simulink model "procesor"  (R2020a)
settings: Solver=VariableStepAuto  StartTime=0.0  StopTime=inf  RelTol=1e-3
libraries: simulink_extras x40, commutil2 x3
settings Model: NumberOfSteps=3  EnablePacing=on  Creator=BakuTer  LastModifiedBy=BakuTer
settings ModelReferenceCC: UpdateModelReferenceTargets=AssumeUpToDate

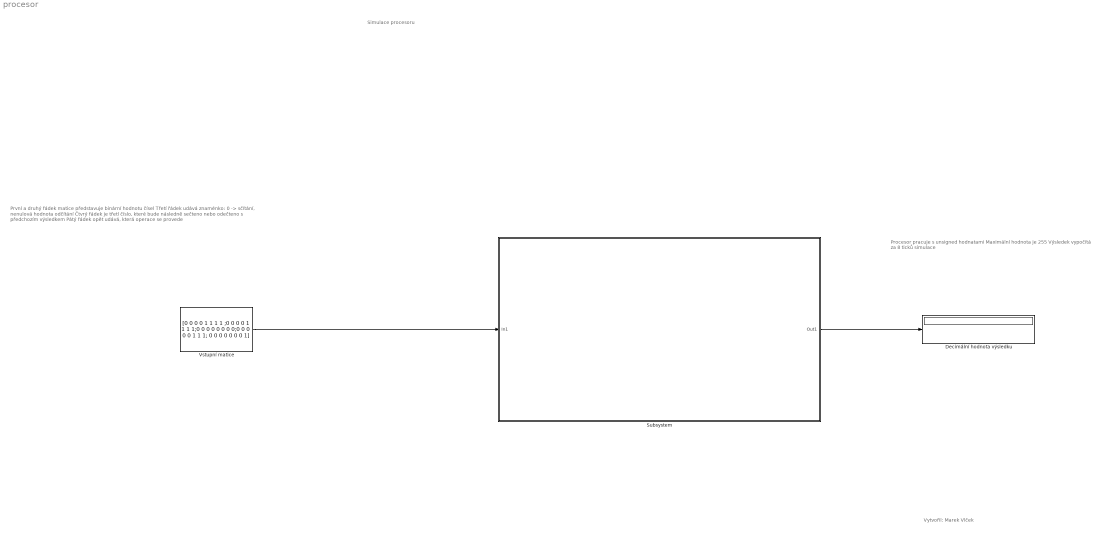
== system procesor ==
  note: Vytvořil: Marek Vlček
  note: Simulace procesoru
  note: Procesor pracuje s unsigned hodnatami
      |
      | Maximální hodnota je 255
      |
      | Výsledek vypočítá za 8 ticků simulace
  note: První a druhý řádek matice představuje binární hodnotu čísel
      |
      | Třetí řádek udává znaménko: 0 -> sčítání, nenulová hodnota odčítání
      |
      | Čtvrý řádek je třetí číslo, které bude následně sečteno nebo odečteno s předchozím výsledkem
      |
      | Pátý řádek opět udává, která operace se provede
  Decimální hodnota výsledku : Display
  Subsystem : Subsystem
      mask Display: image('T:\Stažené Soubory\jak-vybrat-procesor.jpg'); % Use "Edit Image" on toolstrip to change.
  Vstupní matice : Constant  Value=[0 0 0 0 1 1 1 1 ;0 0 0 0 1 1 1 1;0 0 0 0 0 0 0 0;0 0 0 0 0 1 1 1; 0 0 0 0 0 0 0 1]  VectorParams1D=off
  wires:
  Vstupní matice/1 -> Subsystem/1(In1)
  Subsystem/1(Out1) -> Decimální hodnota výsledku/1

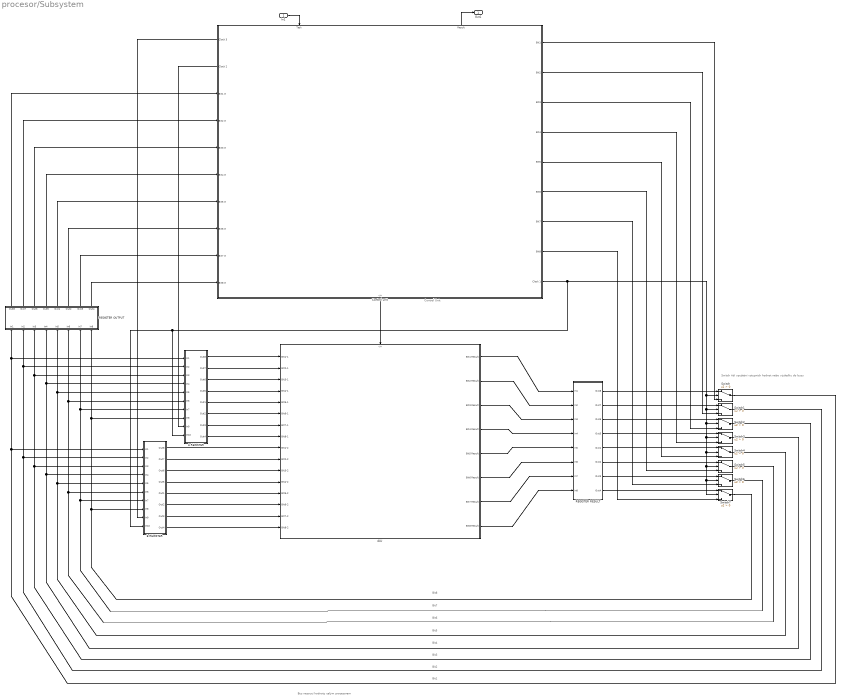
== system procesor/Subsystem ==
  note: Switch řídí vpuštění vstupních hodnot nebo výsledku do busu
  note: Bus nesoucí hodnoty celým procesorem
  note: Bit1
  note: Control Unit
  note: Bit2
  note: Bit3
  note: Bit4
  note: Bit5
  note: Bit6
  note: Bit7
  note: Bit8
  In1 : Inport
  "A REGISTER " : Subsystem
  ALU : Subsystem
      settings: PortSchema="{\"entries\":[{\"content\":{\"sides\":[{\"content\":{\"connectorIds\":[\"In1\",\"In2\",\"In3\",\"In4\",\"In5\",\"In6\",\"In7\",\"In8\",\"In9\",\"In10\",\"In11\",\"In12\",\"In13\",\"In14\",\"In15\",\"In16\"]},\"type\":\"ConnectorPlacement.EquallySpacedRectSide\",\"uuid\":\"ebc9eafb-b3d6-44c3-afac-e365ab2b3d65\"},{\"content\":{\"connectorIds\":[\"Out1\",\"Out2\",\"Out3\",\"Out4\",\"Out5\",\"Out6\",\"Out7\",\"Out8\"],\"side\":\"RIGHT\"},\"type\":\"ConnectorPlacement.EquallySpacedRectSide\",\"uuid\":\"9653c2f1-04bb-448f-a78f-504bc47adb0d\"},{\"content\":{\"connectorIds\":[\"In17\"],\"side\":\"TOP\"},\"type\":\"ConnectorPlacement.EquallySpacedRectSide\",\"uuid\":\"4b4c1363-efa0-4666-9ae9-c7b80d9168bd\"}]},\"type\":\"ConnectorPlacement.EquallySpacedConnector\",\"uuid\":\"b9b0fe66-7efa-45ab-a891-884508afc9d3\"}],\"packageUris\":[\"http://schema.mathworks.com/mf0/Connector/19700101\"],\"version\":\"1.0\"}"
  "B REGISTER " : Subsystem
  Control unit : Subsystem
      settings: PortSchema="{\"entries\":[{\"content\":{\"sides\":[{\"content\":{\"connectorIds\":[\"Out12\",\"Out13\",\"In1\",\"In2\",\"In3\",\"In4\",\"In5\",\"In6\",\"In7\",\"In8\"]},\"type\":\"ConnectorPlacement.EquallySpacedRectSide\",\"uuid\":\"83bcb533-41cd-4a45-82b0-e1e863155d62\"},{\"content\":{\"connectorIds\":[\"Out1\",\"Out2\",\"Out3\",\"Out4\",\"Out5\",\"Out6\",\"Out7\",\"Out8\",\"Out9\"],\"side\":\"RIGHT\"},\"type\":\"ConnectorPlacement.EquallySpacedRectSide\",\"uuid\":\"5279903c-db3c-41cc-9a95-b325bef2964f\"},{\"content\":{\"connectorIds\":[\"In9\",\"Out11\"],\"side\":\"TOP\"},\"type\":\"ConnectorPlacement.EquallySpacedRectSide\",\"uuid\":\"7ad9fff0-61c8-4fe7-a492-4231851eacd1\"},{\"content\":{\"connectorIds\":[\"Out10\"],\"side\":\"BOTTOM\"},\"type\":\"ConnectorPlacement.EquallySpacedRectSide\",\"uuid\":\"4f77aa59-d7ef-4985-b89c-d7e6d2465284\"}]},\"type\":\"ConnectorPlacement.EquallySpacedConnector\",\"uuid\":\"61151066-d116-425f-b948-57ee4dd34c87\"}],\"packageUris\":[\"http://schema.mathworks.com/mf0/Connector/19700101\"],\"version\":\"1.0\"}"
  REGISTER OUTPUT : Subsystem
  "REGISTER RESULT " : Subsystem
  Switch{,1..7} (8 alike) : Switch  Criteria=u2 > Threshold
  Out1 : Outport
  wires:
  Control unit/9(Clock 1) -> Switch2/2, Switch7/2, Switch6/2, Switch5/2, Switch4/2, Switch3/2, Switch1/2, Switch/2, "A REGISTER "/10(In10), "B REGISTER "/10(In10)
  ALU/7(Bit7 Result) -> "REGISTER RESULT "/7(In7)
  Switch2/1 -> "B REGISTER "/3(In3), REGISTER OUTPUT/3(In3), "A REGISTER "/3(In3)
  Control unit/8(Bit8) -> Switch7/3
  REGISTER OUTPUT/4(Out5) -> Control unit/4(Bit4 in)
  ALU/8(Bit8 Result) -> "REGISTER RESULT "/8(In8)
  "A REGISTER "/4(Out5) -> ALU/4(Bit4-1)
  REGISTER OUTPUT/7(Out3) -> Control unit/7(Bit7 in)
  Switch7/1 -> REGISTER OUTPUT/8(In8), "A REGISTER "/8(In8), "B REGISTER "/8(In8)
  "A REGISTER "/3(Out6) -> ALU/3(Bit3-1)
  "REGISTER RESULT "/6(Out2) -> Switch5/1
  ALU/1(Bit1 Result) -> "REGISTER RESULT "/1(In1)
  REGISTER OUTPUT/3(Out6) -> Control unit/3(Bit3 in)
  "B REGISTER "/5(Out1) -> ALU/13(Bit5-2)
  "A REGISTER "/2(Out7) -> ALU/2(Bit2-1)
  "REGISTER RESULT "/3(Out6) -> Switch2/1
  ALU/4(Bit4 Result) -> "REGISTER RESULT "/4(In4)
  "REGISTER RESULT "/4(Out5) -> Switch3/1
  "A REGISTER "/7(Out3) -> ALU/7(Bit7-1)
  "B REGISTER "/1(Out8) -> ALU/9(Bit1-2)
  Switch/1 -> REGISTER OUTPUT/1(In1), "A REGISTER "/1(In1), "B REGISTER "/1(In1)
  Control unit/2(Bit2) -> Switch1/3
  "B REGISTER "/3(Out6) -> ALU/11(Bit3-2)
  "REGISTER RESULT "/7(Out3) -> Switch6/1
  "A REGISTER "/1(Out8) -> ALU/1(Bit1-1)
  Switch1/1 -> REGISTER OUTPUT/2(In2), "A REGISTER "/2(In2), "B REGISTER "/2(In2)
  ALU/2(Bit2 Result) -> "REGISTER RESULT "/2(In2)
  "REGISTER RESULT "/1(Out8) -> Switch/1
  ALU/6(Bit6 Result) -> "REGISTER RESULT "/6(In6)
  "B REGISTER "/6(Out2) -> ALU/14(Bit6-2)
  "B REGISTER "/8(Out4) -> ALU/16(Bit8-2)
  "B REGISTER "/7(Out3) -> ALU/15(Bit7-2)
  "A REGISTER "/8(Out4) -> ALU/8(Bit8-1)
  ALU/3(Bit3 Result) -> "REGISTER RESULT "/3(In3)
  Switch5/1 -> REGISTER OUTPUT/6(In6), "A REGISTER "/6(In6), "B REGISTER "/6(In6)
  "REGISTER RESULT "/8(Out4) -> Switch7/1
  Control unit/5(Bit5) -> Switch4/3
  "A REGISTER "/6(Out2) -> ALU/6(Bit6-1)
  REGISTER OUTPUT/2(Out7) -> Control unit/2(Bit2 in)
  Switch3/1 -> "B REGISTER "/4(In4), "A REGISTER "/4(In4), REGISTER OUTPUT/4(In4)
  "B REGISTER "/2(Out7) -> ALU/10(Bit2-2)
  Control unit/1(Bit1) -> Switch/3
  Control unit/3(Bit3) -> Switch2/3
  Switch6/1 -> REGISTER OUTPUT/7(In7), "A REGISTER "/7(In7), "B REGISTER "/7(In7)
  ALU/5(Bit5 Result) -> "REGISTER RESULT "/5(In5)
  REGISTER OUTPUT/6(Out2) -> Control unit/6(Bit6 in)
  "REGISTER RESULT "/5(Out1) -> Switch4/1
  Control unit/7(Bit7) -> Switch6/3
  Switch4/1 -> REGISTER OUTPUT/5(In5), "A REGISTER "/5(In5), "B REGISTER "/5(In5)
  Control unit/4(Bit4) -> Switch3/3
  REGISTER OUTPUT/1(Out8) -> Control unit/1(Bit1 in)
  In1/1 -> Control unit/9(Task)
  "REGISTER RESULT "/2(Out7) -> Switch1/1
  REGISTER OUTPUT/5(Out1) -> Control unit/5(Bit5 in)
  Control unit/6(Bit6) -> Switch5/3
  Control unit/10(-/+) -> ALU/17(-/+)
  REGISTER OUTPUT/8(Out4) -> Control unit/8(Bit8 in)
  "B REGISTER "/4(Out5) -> ALU/12(Bit4-2)
  Control unit/13(Clock 2) -> "A REGISTER "/9(In9)
  Control unit/12(Clock 3) -> "B REGISTER "/9(In9)
  "A REGISTER "/5(Out1) -> ALU/5(Bit5-1)
  Control unit/11(Result) -> Out1/1

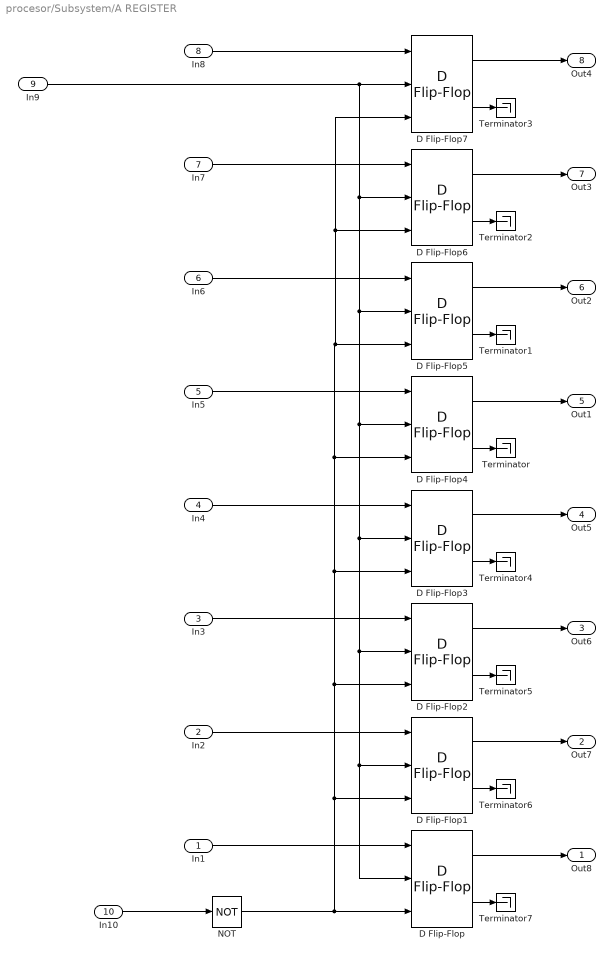
== system procesor/Subsystem/A REGISTER  ==
  In1 : Inport
  In2 : Inport  Port=2
  In3 : Inport  Port=3
  In4 : Inport  Port=4
  In5 : Inport  Port=5
  In6 : Inport  Port=6
  In7 : Inport  Port=7
  In8 : Inport  Port=8
  In9 : Inport  Port=9
  In10 : Inport  Port=10
  D Flip-Flop{,1..7} (8 alike) : simulink_extras/Flip Flops/D Flip-Flop
  NOT : Logic  Operator=NOT  IconShape=distinctive  AllPortsSameDT=off  OutDataTypeStr=boolean
  Terminator{,1..7} (8 alike) : Terminator
  Out8 : Outport
  Out7 : Outport  Port=2
  Out6 : Outport  Port=3
  Out5 : Outport  Port=4
  Out1 : Outport  Port=5
  Out2 : Outport  Port=6
  Out3 : Outport  Port=7
  Out4 : Outport  Port=8
  wires:
  D Flip-Flop5/2 -> Terminator1/1
  D Flip-Flop4/2 -> Terminator/1
  D Flip-Flop5/1 -> Out2/1
  D Flip-Flop3/2 -> Terminator4/1
  In1/1 -> D Flip-Flop/1
  D Flip-Flop6/2 -> Terminator2/1
  D Flip-Flop6/1 -> Out3/1
  D Flip-Flop/1 -> Out8/1
  D Flip-Flop7/2 -> Terminator3/1
  D Flip-Flop2/2 -> Terminator5/1
  D Flip-Flop1/2 -> Terminator6/1
  D Flip-Flop/2 -> Terminator7/1
  D Flip-Flop1/1 -> Out7/1
  D Flip-Flop4/1 -> Out1/1
  D Flip-Flop7/1 -> Out4/1
  In5/1 -> D Flip-Flop4/1
  In3/1 -> D Flip-Flop2/1
  In2/1 -> D Flip-Flop1/1
  In8/1 -> D Flip-Flop7/1
  In6/1 -> D Flip-Flop5/1
  In7/1 -> D Flip-Flop6/1
  In4/1 -> D Flip-Flop3/1
  In9/1 -> D Flip-Flop7/2, D Flip-Flop6/2, D Flip-Flop5/2, D Flip-Flop4/2, D Flip-Flop3/2, D Flip-Flop2/2, D Flip-Flop1/2, D Flip-Flop/2
  D Flip-Flop2/1 -> Out6/1
  D Flip-Flop3/1 -> Out5/1
  In10/1 -> NOT/1
  NOT/1 -> D Flip-Flop/3, D Flip-Flop1/3, D Flip-Flop2/3, D Flip-Flop3/3, D Flip-Flop4/3, D Flip-Flop5/3, D Flip-Flop7/3, D Flip-Flop6/3

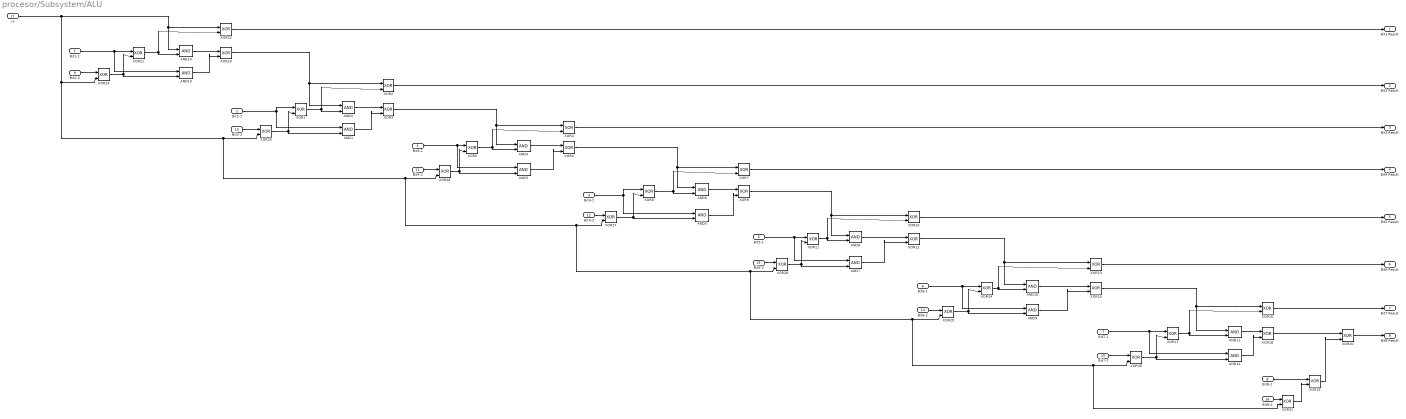
== system procesor/Subsystem/ALU ==
  Bit1-1 : Inport
  Bit2-1 : Inport  Port=2
  Bit3-1 : Inport  Port=3
  Bit4-1 : Inport  Port=4
  Bit5-1 : Inport  Port=5
  Bit6-1 : Inport  Port=6
  Bit7-1 : Inport  Port=7
  Bit8-1 : Inport  Port=8
  Bit1-2 : Inport  Port=9
  Bit2-2 : Inport  Port=10
  Bit3-2 : Inport  Port=11
  Bit4-2 : Inport  Port=12
  Bit5-2 : Inport  Port=13
  Bit6-2 : Inport  Port=14
  Bit7-2 : Inport  Port=15
  Bit8-2 : Inport  Port=16
  -/+ : Inport  Port=17
  AND{1..14} (14 alike) : Logic  IconShape=distinctive  AllPortsSameDT=off  OutDataTypeStr=boolean
  XOR{1..31} (31 alike) : Logic  Operator=XOR  IconShape=distinctive  AllPortsSameDT=off  OutDataTypeStr=boolean
  Bit1 Result : Outport
  Bit2 Result : Outport  Port=2
  Bit3 Result : Outport  Port=3
  Bit4 Result : Outport  Port=4
  Bit5 Result : Outport  Port=5
  Bit6 Result : Outport  Port=6
  Bit7 Result : Outport  Port=7
  Bit8 Result : Outport  Port=8
  wires:
  Bit8-2/1 -> XOR31/1
  XOR21/1 -> XOR22/2, AND14/2
  XOR23/1 -> AND2/1, XOR2/1
  Bit2-1/1 -> XOR1/1, AND1/1
  XOR24/1 -> AND13/2, XOR21/2
  AND14/1 -> XOR23/1
  -/+/1 -> AND14/1, XOR22/1, XOR25/2, XOR27/2, XOR29/2, XOR31/2, XOR30/2, XOR28/2, XOR26/2, XOR24/2
  Bit5-1/1 -> AND7/1, XOR11/1
  Bit7-2/1 -> XOR30/1
  Bit1-2/1 -> XOR24/1
  XOR11/1 -> XOR10/2, AND8/2
  AND6/1 -> XOR9/1
  XOR28/1 -> AND7/2, XOR11/2
  Bit2-2/1 -> XOR25/1
  XOR7/1 -> Bit4 Result/1
  Bit6-1/1 -> AND9/1, XOR14/1
  Bit1-1/1 -> AND13/1, XOR21/1
  Bit4-2/1 -> XOR27/1
  XOR5/1 -> XOR4/2, AND4/2
  XOR13/1 -> Bit6 Result/1
  Bit7-1/1 -> XOR17/1, AND12/1
  Bit8-1/1 -> XOR19/1
  XOR18/1 -> XOR20/1
  XOR27/1 -> XOR8/2, AND5/2
  AND4/1 -> XOR6/1
  XOR22/1 -> Bit1 Result/1
  AND10/1 -> XOR15/1
  AND13/1 -> XOR23/2
  AND11/1 -> XOR18/1
  AND5/1 -> XOR9/2
  Bit5-2/1 -> XOR28/1
  Bit3-2/1 -> XOR26/1
  Bit3-1/1 -> AND3/1, XOR5/1
  XOR9/1 -> XOR10/1, AND8/1
  XOR25/1 -> AND1/2, XOR1/2
  XOR17/1 -> AND11/2, XOR16/2
  Bit4-1/1 -> XOR8/1, AND5/1
  XOR2/1 -> Bit2 Result/1
  XOR29/1 -> AND9/2, XOR14/2
  XOR16/1 -> Bit7 Result/1
  AND2/1 -> XOR3/1
  XOR8/1 -> XOR7/2, AND6/2
  AND1/1 -> XOR3/2
  Bit6-2/1 -> XOR29/1
  XOR3/1 -> AND4/1, XOR4/1
  XOR12/1 -> AND10/1, XOR13/1
  XOR15/1 -> AND11/1, XOR16/1
  XOR26/1 -> AND3/2, XOR5/2
  AND12/1 -> XOR18/2
  XOR1/1 -> XOR2/2, AND2/2
  XOR6/1 -> AND6/1, XOR7/1
  XOR19/1 -> XOR20/2
  AND8/1 -> XOR12/1
  AND7/1 -> XOR12/2
  AND9/1 -> XOR15/2
  XOR20/1 -> Bit8 Result/1
  XOR30/1 -> AND12/2, XOR17/2
  XOR14/1 -> XOR13/2, AND10/2
  AND3/1 -> XOR6/2
  XOR31/1 -> XOR19/2
  XOR4/1 -> Bit3 Result/1
  XOR10/1 -> Bit5 Result/1

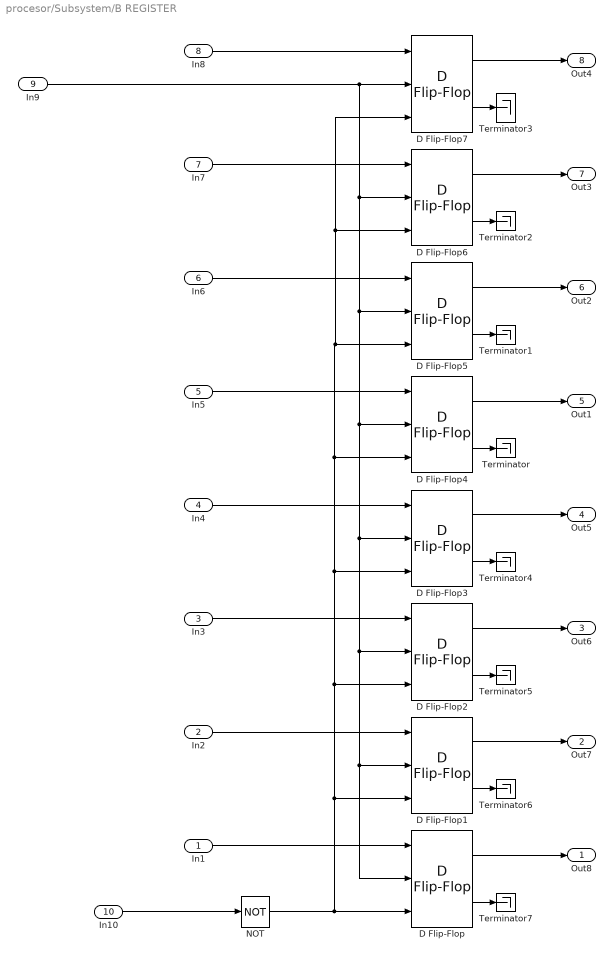
== system procesor/Subsystem/B REGISTER  ==
  In1 : Inport
  In2 : Inport  Port=2
  In3 : Inport  Port=3
  In4 : Inport  Port=4
  In5 : Inport  Port=5
  In6 : Inport  Port=6
  In7 : Inport  Port=7
  In8 : Inport  Port=8
  In9 : Inport  Port=9
  In10 : Inport  Port=10
  D Flip-Flop{,1..7} (8 alike) : simulink_extras/Flip Flops/D Flip-Flop
  NOT : Logic  Operator=NOT  IconShape=distinctive  AllPortsSameDT=off  OutDataTypeStr=boolean
  Terminator{,1..7} (8 alike) : Terminator
  Out8 : Outport
  Out7 : Outport  Port=2
  Out6 : Outport  Port=3
  Out5 : Outport  Port=4
  Out1 : Outport  Port=5
  Out2 : Outport  Port=6
  Out3 : Outport  Port=7
  Out4 : Outport  Port=8
  wires:
  D Flip-Flop3/1 -> Out5/1
  D Flip-Flop2/1 -> Out6/1
  In9/1 -> D Flip-Flop7/2, D Flip-Flop6/2, D Flip-Flop5/2, D Flip-Flop4/2, D Flip-Flop3/2, D Flip-Flop2/2, D Flip-Flop1/2, D Flip-Flop/2
  In4/1 -> D Flip-Flop3/1
  In7/1 -> D Flip-Flop6/1
  In6/1 -> D Flip-Flop5/1
  In8/1 -> D Flip-Flop7/1
  In2/1 -> D Flip-Flop1/1
  In3/1 -> D Flip-Flop2/1
  In5/1 -> D Flip-Flop4/1
  D Flip-Flop7/1 -> Out4/1
  D Flip-Flop4/1 -> Out1/1
  D Flip-Flop1/1 -> Out7/1
  D Flip-Flop/2 -> Terminator7/1
  D Flip-Flop1/2 -> Terminator6/1
  D Flip-Flop2/2 -> Terminator5/1
  D Flip-Flop7/2 -> Terminator3/1
  D Flip-Flop/1 -> Out8/1
  D Flip-Flop6/1 -> Out3/1
  D Flip-Flop6/2 -> Terminator2/1
  In1/1 -> D Flip-Flop/1
  D Flip-Flop3/2 -> Terminator4/1
  D Flip-Flop5/1 -> Out2/1
  D Flip-Flop4/2 -> Terminator/1
  D Flip-Flop5/2 -> Terminator1/1
  In10/1 -> NOT/1
  NOT/1 -> D Flip-Flop/3, D Flip-Flop1/3, D Flip-Flop2/3, D Flip-Flop3/3, D Flip-Flop4/3, D Flip-Flop5/3, D Flip-Flop6/3, D Flip-Flop7/3

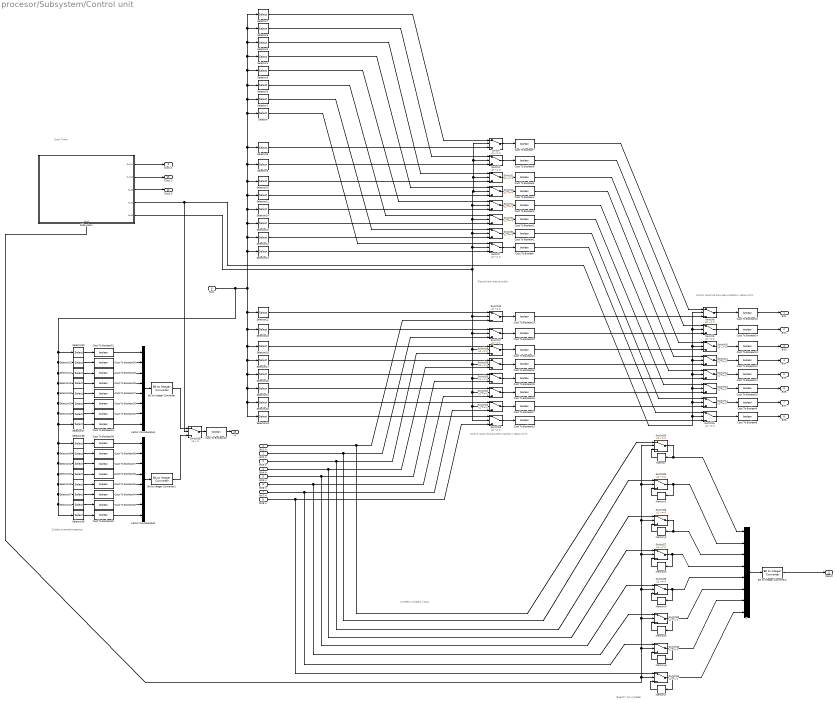
== system procesor/Subsystem/Control unit ==
  note: Switch vpustí do busu jednu hodnotu v danou chvíli
  note: Zjištění znaménka operace
  note: "Registr" pro výsledek
  note: Vyvedení výsledku z busu
  note: Převod čísel matice na bity
  note: Clock Timer
  note: Switch vpustí do busu jednu hodnotu v danou chvíli
  Bit1 in : Inport
  Bit2 in : Inport  Port=2
  Bit3 in : Inport  Port=3
  Bit4 in : Inport  Port=4
  Bit5 in : Inport  Port=5
  Bit6 in : Inport  Port=6
  Bit7 in : Inport  Port=7
  Bit8 in : Inport  Port=8
  Task : Inport  Port=9
  1 : Concatenate  NumInputs=8
  Bit to Integer Converter : commutil2/Bit to Integer Converter  nbits=8  bitOrder=MSB first  signedOutputValues=Signed  outDtype=Inherit via internal rule  outDtypeSigned=Inherit via internal rule
  Bit to Integer Converter1 : commutil2/Bit to Integer Converter  nbits=8  bitOrder=MSB first  signedOutputValues=Signed  outDtype=Inherit via internal rule  outDtypeSigned=Inherit via internal rule
  Bit to Integer Converter2 : commutil2/Bit to Integer Converter  nbits=8  bitOrder=LSB first  signedOutputValues=Unsigned  outDtype=Inherit via internal rule  outDtypeSigned=Inherit via internal rule
  Cast To Boolean{,1..40} (41 alike) : DataTypeConversion  OutDataTypeStr=boolean
  Memory{,1..7} (8 alike) : Memory
  Selector : Selector  NumberOfDimensions=2  InputPortWidth=3  IndexOptions=Starting index (dialog),Starting index (dialog)  Indices=2,1  OutputSizes=1,1
  Selector1 : Selector  NumberOfDimensions=2  InputPortWidth=3  IndexOptions=Starting index (dialog),Starting index (dialog)  Indices=2,2  OutputSizes=1,1
  Selector10 : Selector  NumberOfDimensions=2  InputPortWidth=3  IndexOptions=Starting index (dialog),Starting index (dialog)  Indices=1,6  OutputSizes=1,1
  Selector11 : Selector  NumberOfDimensions=2  InputPortWidth=3  IndexOptions=Starting index (dialog),Starting index (dialog)  Indices=1,5  OutputSizes=1,1
  Selector12 : Selector  NumberOfDimensions=2  InputPortWidth=3  IndexOptions=Starting index (dialog),Starting index (dialog)  Indices=1,2  OutputSizes=1,1
  Selector13 : Selector  NumberOfDimensions=2  InputPortWidth=3  IndexOptions=Starting index (dialog),Starting index (dialog)  Indices=1,1  OutputSizes=1,1
  Selector14 : Selector  NumberOfDimensions=2  InputPortWidth=3  IndexOptions=Starting index (dialog),Starting index (dialog)  Indices=1,4  OutputSizes=1,1
  Selector15 : Selector  NumberOfDimensions=2  InputPortWidth=3  IndexOptions=Starting index (dialog),Starting index (dialog)  Indices=1,3  OutputSizes=1,1
  Selector16 : Selector  NumberOfDimensions=2  InputPortWidth=3  IndexOptions=Starting index (dialog),Starting index (dialog)  Indices=4,6  OutputSizes=1,1
  Selector17 : Selector  NumberOfDimensions=2  InputPortWidth=3  IndexOptions=Starting index (dialog),Starting index (dialog)  Indices=4,5  OutputSizes=1,1
  Selector18 : Selector  NumberOfDimensions=2  InputPortWidth=3  IndexOptions=Starting index (dialog),Starting index (dialog)  Indices=4,2  OutputSizes=1,1
  Selector19 : Selector  NumberOfDimensions=2  InputPortWidth=3  IndexOptions=Starting index (dialog),Starting index (dialog)  Indices=4,1  OutputSizes=1,1
  Selector2 : Selector  NumberOfDimensions=2  InputPortWidth=3  IndexOptions=Starting index (dialog),Starting index (dialog)  Indices=2,3  OutputSizes=1,1
  Selector20 : Selector  NumberOfDimensions=2  InputPortWidth=3  IndexOptions=Starting index (dialog),Starting index (dialog)  Indices=4,4  OutputSizes=1,1
  Selector21 : Selector  NumberOfDimensions=2  InputPortWidth=3  IndexOptions=Starting index (dialog),Starting index (dialog)  Indices=4,3  OutputSizes=1,1
  Selector22 : Selector  NumberOfDimensions=2  InputPortWidth=3  IndexOptions=Starting index (dialog),Starting index (dialog)  Indices=4,8  OutputSizes=1,1
  Selector23 : Selector  NumberOfDimensions=2  InputPortWidth=3  IndexOptions=Starting index (dialog),Starting index (dialog)  Indices=4,7  OutputSizes=1,1
  Selector24 : Selector  NumberOfDimensions=2  InputPortWidth=3  IndexOptions=Starting index (dialog),Starting index (dialog)  Indices=3,3  OutputSizes=1,1
  Selector25 : Selector  NumberOfDimensions=2  InputPortWidth=3  IndexOptions=Starting index (dialog),Starting index (dialog)  Indices=3,4  OutputSizes=1,1
  Selector26 : Selector  NumberOfDimensions=2  InputPortWidth=3  IndexOptions=Starting index (dialog),Starting index (dialog)  Indices=3,7  OutputSizes=1,1
  Selector27 : Selector  NumberOfDimensions=2  InputPortWidth=3  IndexOptions=Starting index (dialog),Starting index (dialog)  Indices=3,8  OutputSizes=1,1
  Selector28 : Selector  NumberOfDimensions=2  InputPortWidth=3  IndexOptions=Starting index (dialog),Starting index (dialog)  Indices=3,5  OutputSizes=1,1
  Selector29 : Selector  NumberOfDimensions=2  InputPortWidth=3  IndexOptions=Starting index (dialog),Starting index (dialog)  Indices=3,6  OutputSizes=1,1
  Selector3 : Selector  NumberOfDimensions=2  InputPortWidth=3  IndexOptions=Starting index (dialog),Starting index (dialog)  Indices=2,4  OutputSizes=1,1
  Selector30 : Selector  NumberOfDimensions=2  InputPortWidth=3  IndexOptions=Starting index (dialog),Starting index (dialog)  Indices=3,1  OutputSizes=1,1
  Selector31 : Selector  NumberOfDimensions=2  InputPortWidth=3  IndexOptions=Starting index (dialog),Starting index (dialog)  Indices=3,2  OutputSizes=1,1
  Selector32 : Selector  NumberOfDimensions=2  InputPortWidth=3  IndexOptions=Starting index (dialog),Starting index (dialog)  Indices=5,3  OutputSizes=1,1
  Selector33 : Selector  NumberOfDimensions=2  InputPortWidth=3  IndexOptions=Starting index (dialog),Starting index (dialog)  Indices=5,4  OutputSizes=1,1
  Selector34 : Selector  NumberOfDimensions=2  InputPortWidth=3  IndexOptions=Starting index (dialog),Starting index (dialog)  Indices=5,7  OutputSizes=1,1
  Selector35 : Selector  NumberOfDimensions=2  InputPortWidth=3  IndexOptions=Starting index (dialog),Starting index (dialog)  Indices=5,8  OutputSizes=1,1
  Selector36 : Selector  NumberOfDimensions=2  InputPortWidth=3  IndexOptions=Starting index (dialog),Starting index (dialog)  Indices=5,5  OutputSizes=1,1
  Selector37 : Selector  NumberOfDimensions=2  InputPortWidth=3  IndexOptions=Starting index (dialog),Starting index (dialog)  Indices=5,6  OutputSizes=1,1
  Selector38 : Selector  NumberOfDimensions=2  InputPortWidth=3  IndexOptions=Starting index (dialog),Starting index (dialog)  Indices=5,1  OutputSizes=1,1
  Selector39 : Selector  NumberOfDimensions=2  InputPortWidth=3  IndexOptions=Starting index (dialog),Starting index (dialog)  Indices=5,2  OutputSizes=1,1
  Selector4 : Selector  NumberOfDimensions=2  InputPortWidth=3  IndexOptions=Starting index (dialog),Starting index (dialog)  Indices=2,5  OutputSizes=1,1
  Selector5 : Selector  NumberOfDimensions=2  InputPortWidth=3  IndexOptions=Starting index (dialog),Starting index (dialog)  Indices=2,6  OutputSizes=1,1
  Selector6 : Selector  NumberOfDimensions=2  InputPortWidth=3  IndexOptions=Starting index (dialog),Starting index (dialog)  Indices=2,7  OutputSizes=1,1
  Selector7 : Selector  NumberOfDimensions=2  InputPortWidth=3  IndexOptions=Starting index (dialog),Starting index (dialog)  Indices=2,8  OutputSizes=1,1
  Selector8 : Selector  NumberOfDimensions=2  InputPortWidth=3  IndexOptions=Starting index (dialog),Starting index (dialog)  Indices=1,8  OutputSizes=1,1
  Selector9 : Selector  NumberOfDimensions=2  InputPortWidth=3  IndexOptions=Starting index (dialog),Starting index (dialog)  Indices=1,7  OutputSizes=1,1
  Subsystem : Subsystem
      settings: PortSchema="{\"entries\":[{\"content\":{\"sides\":[{\"content\":{\"connectorIds\":[]},\"type\":\"ConnectorPlacement.EquallySpacedRectSide\",\"uuid\":\"4b9fa410-50dc-473f-8ff5-bc88434c8eb2\"},{\"content\":{\"connectorIds\":[\"Out1\",\"Out2\",\"Out3\",\"Out4\",\"Out5\"],\"side\":\"RIGHT\"},\"type\":\"ConnectorPlacement.EquallySpacedRectSide\",\"uuid\":\"992e7115-2d07-4769-8824-ecca453ee14e\"},{\"content\":{\"connectorIds\":[],\"side\":\"TOP\"},\"type\":\"ConnectorPlacement.EquallySpacedRectSide\",\"uuid\":\"783a8de9-2d17-4ff6-9655-2506de03f07b\"},{\"content\":{\"connectorIds\":[\"Out6\"],\"side\":\"BOTTOM\"},\"type\":\"ConnectorPlacement.EquallySpacedRectSide\",\"uuid\":\"131e71d1-867a-4410-92f0-a0d2960fd7de\"}]},\"type\":\"ConnectorPlacement.EquallySpacedConnector\",\"uuid\":\"c8c3b98b-9c82-46bc-8b11-ec22577b31ce\"}],\"packageUris\":[\"http://schema.mathworks.com/mf0/Connector/19700101\"],\"version\":\"1.0\"}"
  Switch{,1..27,29..32} (32 alike) : Switch  Criteria=u2 ~= 0
  Switch28 : Switch  Criteria=u2 > Threshold  OutDataTypeStr=int8
  Vector Concatenate1 : Concatenate  NumInputs=8
  Vector Concatenate2 : Concatenate  NumInputs=8
  Bit1 : Outport
  Bit2 : Outport  Port=2
  Bit3 : Outport  Port=3
  Bit4 : Outport  Port=4
  Bit5 : Outport  Port=5
  Bit6 : Outport  Port=6
  Bit7 : Outport  Port=7
  Bit8 : Outport  Port=8
  Clock 1 : Outport  Port=9
  -/+ : Outport  Port=10
  Result : Outport  Port=11
  Clock 3 : Outport  Port=12
  Clock 2 : Outport  Port=13
  wires:
  Switch/1 -> Cast To Boolean7/1
  Switch1/1 -> Cast To Boolean6/1
  Switch2/1 -> Cast To Boolean5/1
  Switch3/1 -> Cast To Boolean4/1
  Switch4/1 -> Cast To Boolean3/1
  Switch5/1 -> Cast To Boolean2/1
  Switch6/1 -> Cast To Boolean1/1
  Switch7/1 -> Cast To Boolean/1
  Subsystem/5(Out3) -> Switch/2, Switch1/2, Switch2/2, Switch3/2, Switch4/2, Switch5/2, Switch6/2, Switch7/2, Switch16/2, Switch17/2, Switch18/2, Switch19/2, Switch20/2, Switch21/2, Switch22/2, Switch23/2
  Cast To Boolean8/1 -> Bit8/1
  Cast To Boolean9/1 -> Bit7/1
  Cast To Boolean10/1 -> Bit6/1
  Cast To Boolean11/1 -> Bit5/1
  Cast To Boolean12/1 -> Bit4/1
  Cast To Boolean13/1 -> Bit3/1
  Cast To Boolean14/1 -> Bit2/1
  Cast To Boolean15/1 -> Bit1/1
  Switch15/1 -> Cast To Boolean8/1
  Switch14/1 -> Cast To Boolean9/1
  Switch13/1 -> Cast To Boolean10/1
  Switch12/1 -> Cast To Boolean11/1
  Switch11/1 -> Cast To Boolean12/1
  Switch10/1 -> Cast To Boolean13/1
  Switch9/1 -> Cast To Boolean14/1
  Switch8/1 -> Cast To Boolean15/1
  Cast To Boolean7/1 -> Switch8/1
  Cast To Boolean6/1 -> Switch9/1
  Cast To Boolean5/1 -> Switch10/1
  Cast To Boolean4/1 -> Switch11/1
  Cast To Boolean3/1 -> Switch12/1
  Cast To Boolean2/1 -> Switch13/1
  Cast To Boolean1/1 -> Switch14/1
  Cast To Boolean/1 -> Switch15/1
  Switch23/1 -> Cast To Boolean16/1
  Switch22/1 -> Cast To Boolean17/1
  Switch21/1 -> Cast To Boolean18/1
  Switch20/1 -> Cast To Boolean19/1
  Switch19/1 -> Cast To Boolean20/1
  Switch18/1 -> Cast To Boolean21/1
  Switch17/1 -> Cast To Boolean22/1
  Switch16/1 -> Cast To Boolean23/1
  Bit1 in/1 -> Switch24/1, Switch16/3
  Bit2 in/1 -> Switch17/3, Switch25/1
  Bit3 in/1 -> Switch18/3, Switch26/1
  Bit4 in/1 -> Switch19/3, Switch27/1
  Bit5 in/1 -> Switch20/3, Switch29/1
  Bit7 in/1 -> Switch22/3, Switch32/1
  Bit8 in/1 -> Switch23/3, Switch31/1
  Cast To Boolean23/1 -> Switch8/3
  Cast To Boolean22/1 -> Switch9/3
  Cast To Boolean21/1 -> Switch10/3
  Cast To Boolean20/1 -> Switch11/3
  Cast To Boolean19/1 -> Switch12/3
  Cast To Boolean18/1 -> Switch13/3
  Cast To Boolean17/1 -> Switch14/3
  Cast To Boolean16/1 -> Switch15/3
  Switch30/1 -> Memory5/1, 1/6
  Switch27/1 -> Memory3/1, 1/4
  Switch26/1 -> 1/3, Memory2/1
  Switch25/1 -> 1/2, Memory1/1
  Bit6 in/1 -> Switch21/3, Switch30/1
  Switch32/1 -> Memory6/1, 1/7
  Switch31/1 -> 1/8, Memory7/1
  Switch24/1 -> 1/1, Memory/1
  Switch29/1 -> Memory4/1, 1/5
  Memory/1 -> Switch24/3
  Memory1/1 -> Switch25/3
  Memory2/1 -> Switch26/3
  Memory3/1 -> Switch27/3
  Memory4/1 -> Switch29/3
  Memory5/1 -> Switch30/3
  Memory6/1 -> Switch32/3
  Memory7/1 -> Switch31/3
  Selector30/1 -> Cast To Boolean31/1
  Selector27/1 -> Cast To Boolean24/1
  Selector26/1 -> Cast To Boolean25/1
  Selector29/1 -> Cast To Boolean26/1
  Selector28/1 -> Cast To Boolean27/1
  Selector25/1 -> Cast To Boolean28/1
  Selector24/1 -> Cast To Boolean29/1
  Selector31/1 -> Cast To Boolean30/1
  Vector Concatenate1/1 -> Bit to Integer Converter/1
  Cast To Boolean24/1 -> Vector Concatenate1/8
  Cast To Boolean25/1 -> Vector Concatenate1/7
  Cast To Boolean26/1 -> Vector Concatenate1/6
  Cast To Boolean28/1 -> Vector Concatenate1/4
  Cast To Boolean27/1 -> Vector Concatenate1/5
  Cast To Boolean29/1 -> Vector Concatenate1/3
  Cast To Boolean30/1 -> Vector Concatenate1/2
  Cast To Boolean31/1 -> Vector Concatenate1/1
  Bit to Integer Converter1/1 -> Switch28/3
  Cast To Boolean39/1 -> Vector Concatenate2/1
  Cast To Boolean38/1 -> Vector Concatenate2/2
  Cast To Boolean37/1 -> Vector Concatenate2/3
  Cast To Boolean35/1 -> Vector Concatenate2/5
  Cast To Boolean36/1 -> Vector Concatenate2/4
  Cast To Boolean34/1 -> Vector Concatenate2/6
  Cast To Boolean33/1 -> Vector Concatenate2/7
  Cast To Boolean32/1 -> Vector Concatenate2/8
  Vector Concatenate2/1 -> Bit to Integer Converter1/1
  Task/1 -> Selector31/1, Selector24/1, Selector26/1, Selector27/1, Selector38/1, Selector33/1, Selector36/1, Selector37/1, Selector34/1, Selector35/1, Selector32/1, Selector39/1, Selector29/1, Selector28/1, Selector25/1, Selector30/1, Selector23/1, Selector20/1, Selector21/1, Selector19/1, Selector18/1, Selector17/1, Selector16/1, Selector22/1, Selector7/1, Selector6/1, Selector5/1, Selector4/1, Selector3/1, Selector2/1, Selector1/1, Selector/1, Selector8/1, Selector9/1, Selector10/1, Selector11/1, Selector14/1, Selector15/1, Selector12/1, Selector13/1
  Selector39/1 -> Cast To Boolean38/1
  Selector32/1 -> Cast To Boolean37/1
  Selector33/1 -> Cast To Boolean36/1
  Selector36/1 -> Cast To Boolean35/1
  Selector37/1 -> Cast To Boolean34/1
  Selector34/1 -> Cast To Boolean33/1
  Selector35/1 -> Cast To Boolean32/1
  Selector38/1 -> Cast To Boolean39/1
  Switch28/1 -> Cast To Boolean40/1
  Subsystem/4(Out2) -> Switch8/2, Switch9/2, Switch10/2, Switch11/2, Switch12/2, Switch13/2, Switch14/2, Switch15/2, Switch28/2
  Bit to Integer Converter/1 -> Switch28/1
  Subsystem/1(Out11) -> Clock 1/1
  Subsystem/2(Out10) -> Clock 2/1
  Subsystem/3(Out9) -> Clock 3/1
  1/1 -> Bit to Integer Converter2/1
  Selector7/1 -> Switch/1
  Selector6/1 -> Switch1/1
  Selector5/1 -> Switch2/1
  Selector4/1 -> Switch3/1
  Selector3/1 -> Switch4/1
  Selector2/1 -> Switch5/1
  Selector1/1 -> Switch6/1
  Selector/1 -> Switch7/1
  Selector13/1 -> Switch7/3
  Selector12/1 -> Switch6/3
  Selector15/1 -> Switch5/3
  Selector14/1 -> Switch4/3
  Selector11/1 -> Switch3/3
  Selector10/1 -> Switch2/3
  Selector9/1 -> Switch1/3
  Selector8/1 -> Switch/3
  Selector22/1 -> Switch16/1
  Selector23/1 -> Switch17/1
  Selector16/1 -> Switch18/1
  Selector17/1 -> Switch19/1
  Selector20/1 -> Switch20/1
  Selector21/1 -> Switch21/1
  Selector18/1 -> Switch22/1
  Selector19/1 -> Switch23/1
  Subsystem/6(Out1) -> Switch24/2, Switch25/2, Switch26/2, Switch27/2, Switch29/2, Switch30/2, Switch32/2, Switch31/2
  Bit to Integer Converter2/1 -> Result/1
  Cast To Boolean40/1 -> -/+/1

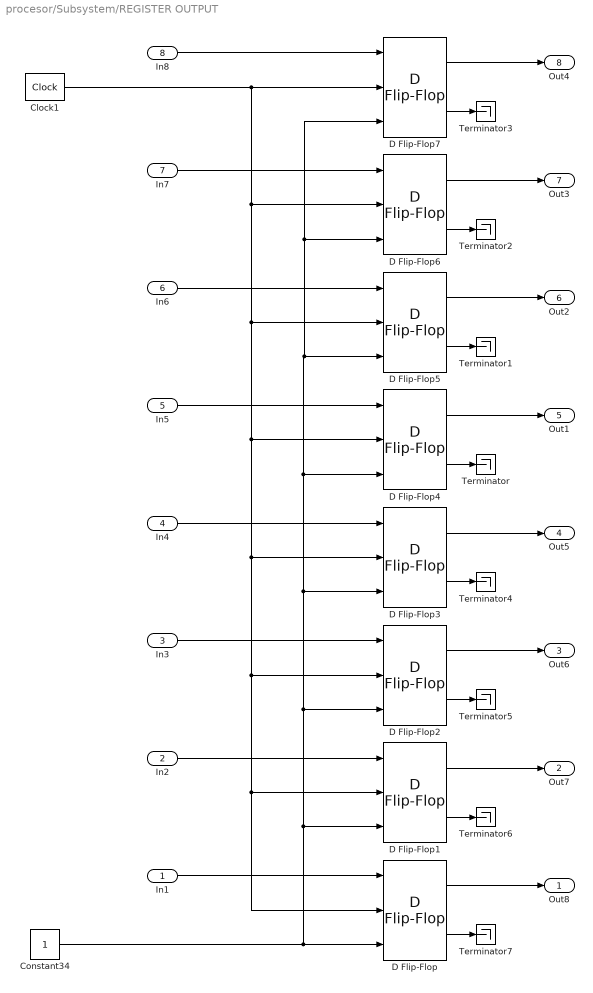
== system procesor/Subsystem/REGISTER OUTPUT ==
  In1 : Inport
  In2 : Inport  Port=2
  In3 : Inport  Port=3
  In4 : Inport  Port=4
  In5 : Inport  Port=5
  In6 : Inport  Port=6
  In7 : Inport  Port=7
  In8 : Inport  Port=8
  Clock1 : simulink_extras/Flip Flops/Clock  period=4
  Constant34 : Constant  OutDataTypeStr=boolean
  D Flip-Flop{,1..7} (8 alike) : simulink_extras/Flip Flops/D Flip-Flop
  Terminator{,1..7} (8 alike) : Terminator
  Out8 : Outport
  Out7 : Outport  Port=2
  Out6 : Outport  Port=3
  Out5 : Outport  Port=4
  Out1 : Outport  Port=5
  Out2 : Outport  Port=6
  Out3 : Outport  Port=7
  Out4 : Outport  Port=8
  wires:
  D Flip-Flop3/1 -> Out5/1
  D Flip-Flop2/1 -> Out6/1
  Clock1/1 -> D Flip-Flop7/2, D Flip-Flop4/2, D Flip-Flop3/2, D Flip-Flop/2, D Flip-Flop1/2, D Flip-Flop2/2, D Flip-Flop5/2, D Flip-Flop6/2
  In4/1 -> D Flip-Flop3/1
  In7/1 -> D Flip-Flop6/1
  In6/1 -> D Flip-Flop5/1
  In8/1 -> D Flip-Flop7/1
  In2/1 -> D Flip-Flop1/1
  In3/1 -> D Flip-Flop2/1
  In5/1 -> D Flip-Flop4/1
  D Flip-Flop7/1 -> Out4/1
  D Flip-Flop4/1 -> Out1/1
  D Flip-Flop1/1 -> Out7/1
  D Flip-Flop/2 -> Terminator7/1
  D Flip-Flop1/2 -> Terminator6/1
  D Flip-Flop2/2 -> Terminator5/1
  D Flip-Flop7/2 -> Terminator3/1
  D Flip-Flop/1 -> Out8/1
  D Flip-Flop6/1 -> Out3/1
  D Flip-Flop6/2 -> Terminator2/1
  In1/1 -> D Flip-Flop/1
  D Flip-Flop3/2 -> Terminator4/1
  D Flip-Flop5/1 -> Out2/1
  D Flip-Flop4/2 -> Terminator/1
  D Flip-Flop5/2 -> Terminator1/1
  Constant34/1 -> D Flip-Flop/3, D Flip-Flop2/3, D Flip-Flop7/3, D Flip-Flop6/3, D Flip-Flop5/3, D Flip-Flop4/3, D Flip-Flop3/3, D Flip-Flop1/3

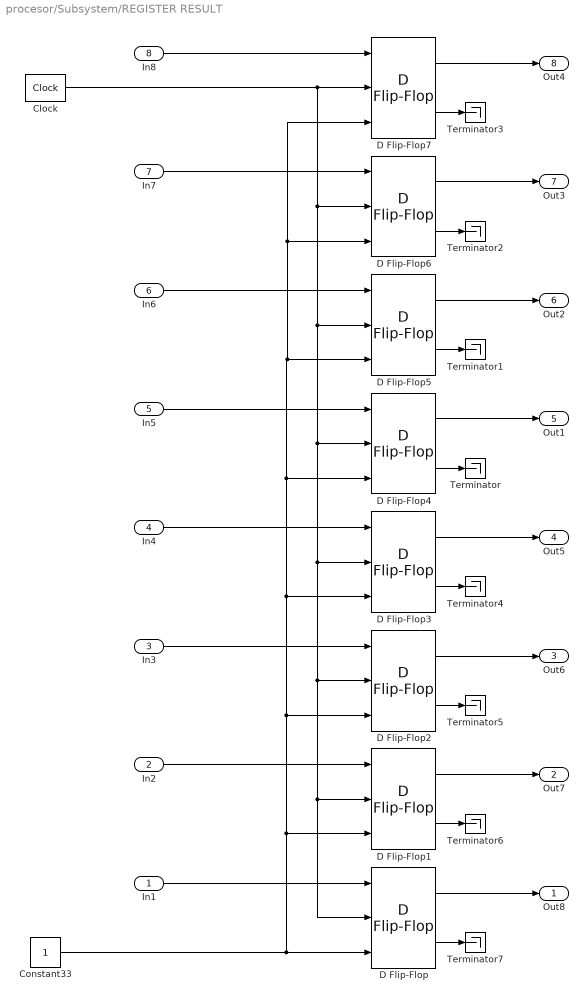
== system procesor/Subsystem/REGISTER RESULT  ==
  In1 : Inport
  In2 : Inport  Port=2
  In3 : Inport  Port=3
  In4 : Inport  Port=4
  In5 : Inport  Port=5
  In6 : Inport  Port=6
  In7 : Inport  Port=7
  In8 : Inport  Port=8
  Clock : simulink_extras/Flip Flops/Clock  period=1
  Constant33 : Constant  OutDataTypeStr=boolean
  D Flip-Flop{,1..7} (8 alike) : simulink_extras/Flip Flops/D Flip-Flop
  Terminator{,1..7} (8 alike) : Terminator
  Out8 : Outport
  Out7 : Outport  Port=2
  Out6 : Outport  Port=3
  Out5 : Outport  Port=4
  Out1 : Outport  Port=5
  Out2 : Outport  Port=6
  Out3 : Outport  Port=7
  Out4 : Outport  Port=8
  wires:
  D Flip-Flop5/2 -> Terminator1/1
  D Flip-Flop4/2 -> Terminator/1
  D Flip-Flop5/1 -> Out2/1
  D Flip-Flop3/2 -> Terminator4/1
  In1/1 -> D Flip-Flop/1
  D Flip-Flop6/2 -> Terminator2/1
  D Flip-Flop6/1 -> Out3/1
  D Flip-Flop/1 -> Out8/1
  D Flip-Flop7/2 -> Terminator3/1
  D Flip-Flop2/2 -> Terminator5/1
  D Flip-Flop1/2 -> Terminator6/1
  D Flip-Flop/2 -> Terminator7/1
  D Flip-Flop1/1 -> Out7/1
  D Flip-Flop4/1 -> Out1/1
  D Flip-Flop7/1 -> Out4/1
  In5/1 -> D Flip-Flop4/1
  In3/1 -> D Flip-Flop2/1
  In2/1 -> D Flip-Flop1/1
  In8/1 -> D Flip-Flop7/1
  In6/1 -> D Flip-Flop5/1
  In7/1 -> D Flip-Flop6/1
  In4/1 -> D Flip-Flop3/1
  Clock/1 -> D Flip-Flop7/2, D Flip-Flop6/2, D Flip-Flop5/2, D Flip-Flop4/2, D Flip-Flop3/2, D Flip-Flop2/2, D Flip-Flop1/2, D Flip-Flop/2
  D Flip-Flop2/1 -> Out6/1
  D Flip-Flop3/1 -> Out5/1
  Constant33/1 -> D Flip-Flop/3, D Flip-Flop1/3, D Flip-Flop2/3, D Flip-Flop3/3, D Flip-Flop4/3, D Flip-Flop5/3, D Flip-Flop7/3, D Flip-Flop6/3

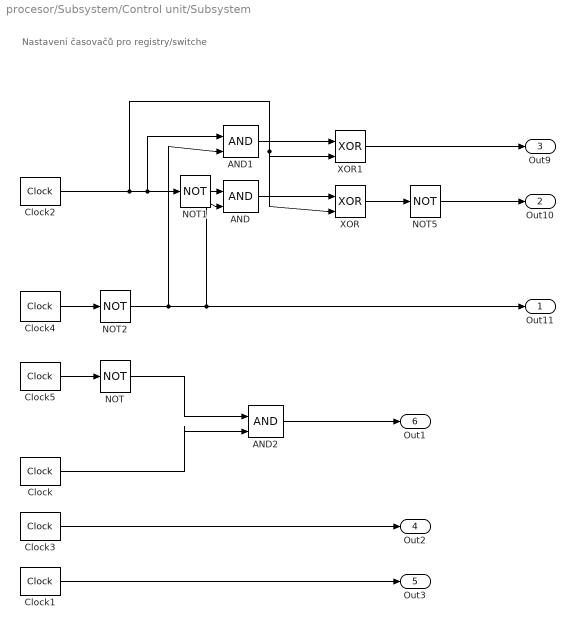
== system procesor/Subsystem/Control unit/Subsystem ==
  note: Nastavení časovačů pro registry/switche
  AND : Logic  IconShape=distinctive  AllPortsSameDT=off  OutDataTypeStr=boolean
  AND1 : Logic  IconShape=distinctive  AllPortsSameDT=off  OutDataTypeStr=boolean
  AND2 : Logic  IconShape=distinctive  AllPortsSameDT=off  OutDataTypeStr=boolean
  Clock : simulink_extras/Flip Flops/Clock  period=8
  Clock1 : simulink_extras/Flip Flops/Clock  period=2
  Clock2 : simulink_extras/Flip Flops/Clock  period=1
  Clock3 : simulink_extras/Flip Flops/Clock  period=8
  Clock4 : simulink_extras/Flip Flops/Clock  period=4
  Clock5 : simulink_extras/Flip Flops/Clock  period=16
  NOT{,1..2,5} (4 alike) : Logic  Operator=NOT  IconShape=distinctive  AllPortsSameDT=off  OutDataTypeStr=boolean
  XOR : Logic  Operator=XOR  IconShape=distinctive  AllPortsSameDT=off  OutDataTypeStr=boolean
  XOR1 : Logic  Operator=XOR  IconShape=distinctive  AllPortsSameDT=off  OutDataTypeStr=boolean
  Out11 : Outport
  Out10 : Outport  Port=2
  Out9 : Outport  Port=3
  Out2 : Outport  Port=4
  Out3 : Outport  Port=5
  Out1 : Outport  Port=6
  wires:
  Clock4/1 -> NOT2/1
  Clock2/1 -> XOR/2, XOR1/2, NOT1/1, AND1/1
  NOT1/1 -> AND/1
  XOR/1 -> NOT5/1
  NOT2/1 -> Out11/1, AND/2, AND1/2
  NOT5/1 -> Out10/1
  AND/1 -> XOR/1
  AND1/1 -> XOR1/1
  XOR1/1 -> Out9/1
  NOT/1 -> AND2/1
  Clock/1 -> AND2/2
  Clock5/1 -> NOT/1
  AND2/1 -> Out1/1
  Clock3/1 -> Out2/1
  Clock1/1 -> Out3/1
